simulink model "SalientPolePMSM"  (R2020b)
settings: Solver=VariableStepAuto  StartTime=0  StopTime=1  MaxStep=1e-4  RelTol=1e-4
values from neighbouring files (symbols this model uses):
  Bgain = 1    [DataSalientPolePMSM-DESKTOP-IINSHMA.m]    (also in DataSalientPolePMSM.m)
  Gcc_1ord = 1/(s/bandwidth(Gcc) + 1)    [DataSalientPolePMSM-DESKTOP-IINSHMA.m]    (also in DataSalientPolePMSM.m)
  lamdVec = mot.Ld*idVec+mot.lammg    [DataSalientPolePMSM-DESKTOP-IINSHMA.m]    (also in DataSalientPolePMSM.m)
  lamqVec = mot.Lq*iqVec    [DataSalientPolePMSM-DESKTOP-IINSHMA.m]    (also in DataSalientPolePMSM.m)
  TAB0_abc = Tabc_AB0^-1    [DataSalientPolePMSM-DESKTOP-IINSHMA.m]    (also in DataSalientPolePMSM.m)
  Tabc_AB0 = 2/3.*[     1       -1/2       -1/2 ... (first row only)    [DataSalientPolePMSM-DESKTOP-IINSHMA.m]    (also in DataSalientPolePMSM.m)
  Talphabeta_abc = Tabc_alphabeta^(-1)    [DataSalientPolePMSM-DESKTOP-IINSHMA.m]    (also in DataSalientPolePMSM.m)
undefined symbols (not defined in the file or in its folder): DiscIntNeverNeededParam, dqpll, inv, kid, kpd, magnitude, meas, mot, Obs, PI, stconv
libraries: simulink x53, pid_lib x3, powerlib x2, eeBldcCommutationLogic x1, electricdrivelib x1
(part 3 of 7)

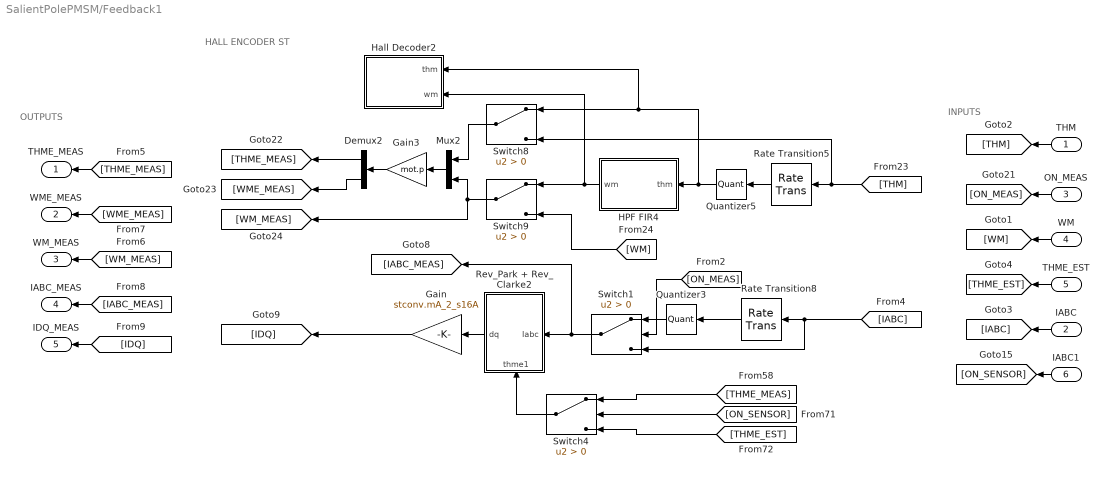
== system SalientPolePMSM/Feedback1 ==
  note: OUTPUTS
  note: INPUTS
  note: HALL ENCODER ST
  THM : Inport
  IABC : Inport  Port=2
  ON_MEAS : Inport  Port=3
  WM : Inport  Port=4
  THME_EST : Inport  Port=5
  IABC1 : Inport  Port=6
  Demux2 : Demux  Outputs=2
  Gain : Gain  Gain=stconv.mA_2_s16A
  Gain3 : Gain  Gain=mot.p
  HPF FIR4 : MATLAB Function  TreatAsAtomicUnit=on
  Hall Decoder2 : Subsystem
  Mux2 : Mux  Inputs=2
  Quantizer3 : Quantizer  QuantizationInterval=meas.cur.adc.q
  Quantizer5 : Quantizer  QuantizationInterval=meas.hall.q
  Rate Transition5 : RateTransition  OutPortSampleTime=meas.hall.Ts
  Rate Transition8 : RateTransition  OutPortSampleTime=inv.Tpwm
  Rev_Park + Rev_Clarke2 : Subsystem
      settings: PortSchema="{\"entries\":[{\"content\":{\"sides\":[{\"content\":{\"connectorIds\":[\"In1\"]},\"type\":\"ConnectorPlacement.EquallySpacedRectSide\",\"uuid\":\"2aae3f04-c402-455e-9a5d-4c573bec95dc\"},{\"content\":{\"connectorIds\":[\"Out1\"],\"side\":\"RIGHT\"},\"type\":\"ConnectorPlacement.EquallySpacedRectSide\",\"uuid\":\"f1532c60-2267-456b-9c2f-34e60e60798d\"},{\"content\":{\"connectorIds\":[],\"side\":\"TOP\"},\"type\":\"ConnectorPlacement.EquallySpacedRectSide\",\"uuid\":\"04e1a6cc-513a-47f7-a63d-759add73a2e3\"},{\"content\":{\"connectorIds\":[\"In2\"],\"side\":\"BOTTOM\"},\"type\":\"ConnectorPlacement.EquallySpacedRectSide\",\"uuid\":\"e4fadd8d-bc98-4107-9436-b30fd69f2e4f\"},{\"content\":{\"connectorIds\":[],\"side\":\"HIDDEN\"},\"type\":\"ConnectorPlacement.EquallySpacedRectSide\",\"uuid\":\"086bd472-9627-4f82-bc83-4764e9943a88\"}]},\"type\":\"ConnectorPlacement.EquallySpacedConnector\",\"uuid\":\"0de85400-6c41-4ce8-8482-fdca09eb4650\"}],\"packageUris\":[\"http://schema.mathworks.com/mf0/Connector/R2020b\"],\"version\":\"1.0\"}"
  Switch{1,4,8..9} (4 alike) : Switch  Criteria=u2 > Threshold
  THME_MEAS : Outport
  WME_MEAS : Outport  Port=2
  WM_MEAS : Outport  Port=3
  IABC_MEAS : Outport  Port=4
  IDQ_MEAS : Outport  Port=5
  wires:
  THME_EST/1 -> [THME_EST]
  WM/1 -> [WM]
  ON_MEAS/1 -> [ON_MEAS]
  Switch1/1 -> Rev_Park + Rev_Clarke2/1(Iabc), [IABC_MEAS]
  [ON_MEAS] -> Switch1/2
  Rate Transition8/1 -> Quantizer3/1
  Quantizer3/1 -> Switch1/1
  THM/1 -> [THM]
  IABC/1 -> [IABC]
  [IABC] -> Switch1/3, Rate Transition8/1
  [THME_MEAS] -> THME_MEAS/1
  [WME_MEAS] -> WME_MEAS/1
  [WM_MEAS] -> WM_MEAS/1
  [IDQ] -> IDQ_MEAS/1
  [IABC_MEAS] -> IABC_MEAS/1
  Rev_Park + Rev_Clarke2/1(dq) -> Gain/1
  IABC1/1 -> [ON_SENSOR]
  [ON_SENSOR] -> Switch4/2
  [WM] -> Switch9/3
  [THM] -> Switch8/3, Rate Transition5/1
  Demux2/2 -> [WME_MEAS]
  Mux2/1 -> Gain3/1
  Gain3/1 -> Demux2/1
  Rate Transition5/1 -> Quantizer5/1
  Switch8/1 -> Mux2/1
  HPF FIR4/1(wm) -> Switch9/1, Hall Decoder2/2(wm)
  Switch9/1 -> Mux2/2, [WM_MEAS]
  Demux2/1 -> [THME_MEAS]
  Quantizer5/1 -> HPF FIR4/1(thm), Hall Decoder2/1(thm), Switch8/1
  Gain/1 -> [IDQ]
  [THME_MEAS] -> Switch4/1
  [THME_EST] -> Switch4/3
  Switch4/1 -> Rev_Park + Rev_Clarke2/2(thme1)

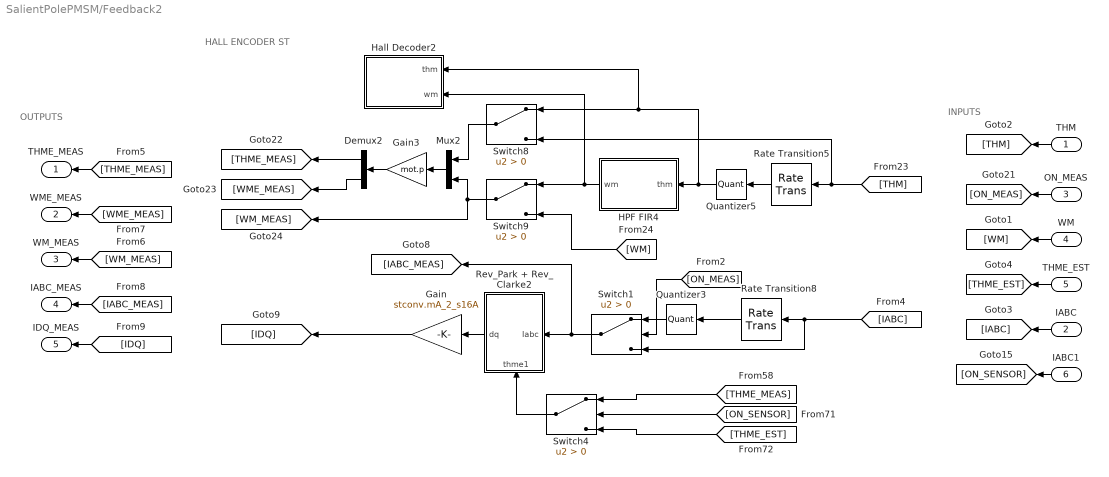
== system SalientPolePMSM/Feedback2 ==
  note: OUTPUTS
  note: INPUTS
  note: HALL ENCODER ST
  THM : Inport
  IABC : Inport  Port=2
  ON_MEAS : Inport  Port=3
  WM : Inport  Port=4
  THME_EST : Inport  Port=5
  IABC1 : Inport  Port=6
  Demux2 : Demux  Outputs=2
  Gain : Gain  Gain=stconv.mA_2_s16A
  Gain3 : Gain  Gain=mot.p
  HPF FIR4 : MATLAB Function  TreatAsAtomicUnit=on
  Hall Decoder2 : Subsystem
  Mux2 : Mux  Inputs=2
  Quantizer3 : Quantizer  QuantizationInterval=meas.cur.adc.q
  Quantizer5 : Quantizer  QuantizationInterval=meas.hall.q
  Rate Transition5 : RateTransition  OutPortSampleTime=meas.hall.Ts
  Rate Transition8 : RateTransition  OutPortSampleTime=inv.Tpwm
  Rev_Park + Rev_Clarke2 : Subsystem
      settings: PortSchema="{\"entries\":[{\"content\":{\"sides\":[{\"content\":{\"connectorIds\":[\"In1\"]},\"type\":\"ConnectorPlacement.EquallySpacedRectSide\",\"uuid\":\"2aae3f04-c402-455e-9a5d-4c573bec95dc\"},{\"content\":{\"connectorIds\":[\"Out1\"],\"side\":\"RIGHT\"},\"type\":\"ConnectorPlacement.EquallySpacedRectSide\",\"uuid\":\"f1532c60-2267-456b-9c2f-34e60e60798d\"},{\"content\":{\"connectorIds\":[],\"side\":\"TOP\"},\"type\":\"ConnectorPlacement.EquallySpacedRectSide\",\"uuid\":\"04e1a6cc-513a-47f7-a63d-759add73a2e3\"},{\"content\":{\"connectorIds\":[\"In2\"],\"side\":\"BOTTOM\"},\"type\":\"ConnectorPlacement.EquallySpacedRectSide\",\"uuid\":\"e4fadd8d-bc98-4107-9436-b30fd69f2e4f\"},{\"content\":{\"connectorIds\":[],\"side\":\"HIDDEN\"},\"type\":\"ConnectorPlacement.EquallySpacedRectSide\",\"uuid\":\"086bd472-9627-4f82-bc83-4764e9943a88\"}]},\"type\":\"ConnectorPlacement.EquallySpacedConnector\",\"uuid\":\"0de85400-6c41-4ce8-8482-fdca09eb4650\"}],\"packageUris\":[\"http://schema.mathworks.com/mf0/Connector/R2020b\"],\"version\":\"1.0\"}"
  Switch{1,4,8..9} (4 alike) : Switch  Criteria=u2 > Threshold
  THME_MEAS : Outport
  WME_MEAS : Outport  Port=2
  WM_MEAS : Outport  Port=3
  IABC_MEAS : Outport  Port=4
  IDQ_MEAS : Outport  Port=5
  wires:
  THME_EST/1 -> [THME_EST]
  WM/1 -> [WM]
  ON_MEAS/1 -> [ON_MEAS]
  Switch1/1 -> Rev_Park + Rev_Clarke2/1(Iabc), [IABC_MEAS]
  [ON_MEAS] -> Switch1/2
  Rate Transition8/1 -> Quantizer3/1
  Quantizer3/1 -> Switch1/1
  THM/1 -> [THM]
  IABC/1 -> [IABC]
  [IABC] -> Switch1/3, Rate Transition8/1
  [THME_MEAS] -> THME_MEAS/1
  [WME_MEAS] -> WME_MEAS/1
  [WM_MEAS] -> WM_MEAS/1
  [IDQ] -> IDQ_MEAS/1
  [IABC_MEAS] -> IABC_MEAS/1
  Rev_Park + Rev_Clarke2/1(dq) -> Gain/1
  IABC1/1 -> [ON_SENSOR]
  [ON_SENSOR] -> Switch4/2
  [WM] -> Switch9/3
  [THM] -> Switch8/3, Rate Transition5/1
  Demux2/2 -> [WME_MEAS]
  Mux2/1 -> Gain3/1
  Gain3/1 -> Demux2/1
  Rate Transition5/1 -> Quantizer5/1
  Switch8/1 -> Mux2/1
  HPF FIR4/1(wm) -> Switch9/1, Hall Decoder2/2(wm)
  Switch9/1 -> Mux2/2, [WM_MEAS]
  Demux2/1 -> [THME_MEAS]
  Quantizer5/1 -> HPF FIR4/1(thm), Hall Decoder2/1(thm), Switch8/1
  Gain/1 -> [IDQ]
  [THME_MEAS] -> Switch4/1
  [THME_EST] -> Switch4/3
  Switch4/1 -> Rev_Park + Rev_Clarke2/2(thme1)

== system SalientPolePMSM/Fuzzy PI ==
  note: INPUTS:
  note: OUTPUT:
  wm* : Inport
  wm : Inport  Port=2
  " " : MATLAB Function  TreatAsAtomicUnit=on
  "  " : MATLAB Function  TreatAsAtomicUnit=on
  "   " : MATLAB Function  TreatAsAtomicUnit=on
  Gain : Gain  Gain=60/(2*3.14)
  Gain1 : Gain  Gain=60/(2*3.14)
  Rule base : MATLAB Function  Commented=on  TreatAsAtomicUnit=on
  Saturation : Saturate  UpperLimit=mot.IN*mot.kTau  LowerLimit=-mot.IN*mot.kTau
  Scope : Scope  NumInputPorts=2
  Scope1 : Scope  NumInputPorts=2
  Sum : Sum  Inputs=|+-
  tau*sat : Outport
  wires:
  "  "/1(isMember) -> Scope1/1, "   "/1(isMember)
  " "/1(isMember_P) -> "  "/1(isMember_P)
  Sum/1 -> " "/1(err)
  Rule base/1(y) -> ?
  " "/4(isNotMember_I) -> "  "/4(isNotMember_I)
  "  "/2(isNotMember) -> Scope1/2, "   "/2(isNotMember)
  " "/2(isNotMember_P) -> "  "/2(isNotMember_P)
  " "/3(isMember_I) -> "  "/3(isMember_I)
  wm*/1 -> Gain/1
  wm/1 -> Gain1/1
  Gain/1 -> Sum/1
  Gain1/1 -> Sum/2
  "   "/1(tau) -> tau*sat/1

== system SalientPolePMSM/Fuzzy PI1 ==
  note: INPUTS:
  note: OUTPUT:
  wm* : Inport
  wm : Inport  Port=2
  " " : MATLAB Function  TreatAsAtomicUnit=on
  "  " : MATLAB Function  TreatAsAtomicUnit=on
  "   " : MATLAB Function  TreatAsAtomicUnit=on
  Rule base : MATLAB Function  Commented=on  TreatAsAtomicUnit=on
  Saturation : Saturate  UpperLimit=10  LowerLimit=-10
  Scope : Scope  NumInputPorts=2
  Scope1 : Scope  NumInputPorts=2
  Sum : Sum  Inputs=|+-
  tau*sat : Outport
  wires:
  "  "/1(isMember) -> Scope1/1, "   "/1(isMember)
  " "/1(isMember_P) -> "  "/1(isMember_P)
  Sum/1 -> " "/1(err)
  Rule base/1(y) -> ?
  " "/4(isNotMember_I) -> "  "/4(isNotMember_I)
  "  "/2(isNotMember) -> Scope1/2, "   "/2(isNotMember)
  " "/2(isNotMember_P) -> "  "/2(isNotMember_P)
  " "/3(isMember_I) -> "  "/3(isMember_I)
  wm*/1 -> Scope/1, Sum/1
  wm/1 -> Scope/2, Sum/2
  Saturation/1 -> tau*sat/1  "tau*sat"
  "   "/1(tau) -> Saturation/1  "tau*"

== system SalientPolePMSM/Fuzzy PI2 ==
  note: INPUTS:
  note: OUTPUT:
  wm* : Inport
  wm : Inport  Port=2
  " " : MATLAB Function  TreatAsAtomicUnit=on
  "  " : MATLAB Function  TreatAsAtomicUnit=on
  "   " : MATLAB Function  TreatAsAtomicUnit=on
  Gain : Gain  Gain=60/(2*3.14)
  Gain1 : Gain  Gain=60/(2*3.14)
  Rule base : MATLAB Function  Commented=on  TreatAsAtomicUnit=on
  Saturation : Saturate  UpperLimit=mot.IN*mot.kTau  LowerLimit=-mot.IN*mot.kTau
  Scope : Scope  NumInputPorts=2
  Scope1 : Scope  NumInputPorts=2
  Sum : Sum  Inputs=|+-
  tau*sat : Outport
  wires:
  "  "/1(isMember) -> Scope1/1, "   "/1(isMember)
  " "/1(isMember_P) -> "  "/1(isMember_P)
  Sum/1 -> " "/1(err)
  Rule base/1(y) -> ?
  " "/4(isNotMember_I) -> "  "/4(isNotMember_I)
  "  "/2(isNotMember) -> Scope1/2, "   "/2(isNotMember)
  " "/2(isNotMember_P) -> "  "/2(isNotMember_P)
  " "/3(isMember_I) -> "  "/3(isMember_I)
  wm*/1 -> Gain/1
  wm/1 -> Gain1/1
  Gain/1 -> Sum/1
  Gain1/1 -> Sum/2
  "   "/1(tau) -> tau*sat/1

== system SalientPolePMSM/INVERTER ==
  note: INPUTS:
  note: OUTPUTS:
  uAB : Inport
  uBus : Inport  Port=2
  iabc : Inport  Port=3
  INVERTER power driver : Subsystem
  SVM algorithm : Subsystem
  uabc_n* : Outport
  uabc_n*nonideal : Outport  Port=2
  satON : Outport  Port=3
  duties : Outport  Port=4
  wires:
  uBus/1 -> SVM algorithm/2(uBus), INVERTER power driver/2(uBus)
  SVM algorithm/2(satON) -> [satON]
  [satON] -> satON/1
  SVM algorithm/1(duties) -> duties/1, INVERTER power driver/1(duties)  "duties"
  iabc/1 -> INVERTER power driver/3(iabc)
  INVERTER power driver/1(uabc_n*) -> uabc_n*/1
  INVERTER power driver/2(uabc_n*nonideal) -> uabc_n*nonideal/1
  uAB/1 -> SVM algorithm/1(UABref)

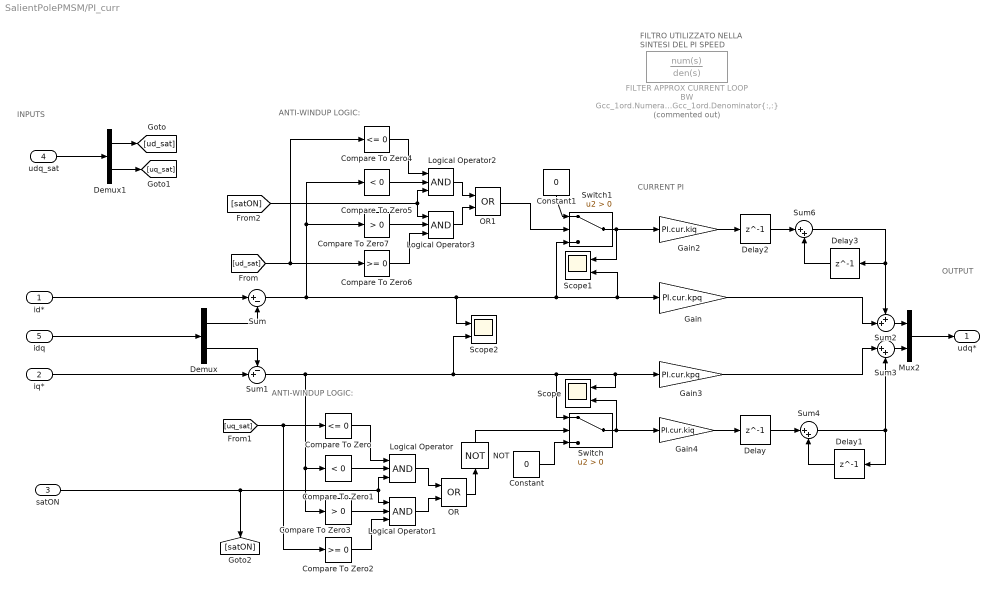
== system SalientPolePMSM/PI_curr ==
  note: FILTRO UTILIZZATO
      | NELLA SINTESI DEL
      | PI SPEED
  note: CURRENT PI
  note: ANTI-WINDUP LOGIC:
  note: ANTI-WINDUP LOGIC:
  note: OUTPUT
  note: INPUTS
  id* : Inport
  iq* : Inport  Port=2
  satON : Inport  Port=3
  udq_sat : Inport  Port=4
  idq : Inport  Port=5
  Compare To Zero : simulink/Logic and Bit Operations/Compare To Zero  relop=<=  OutDataTypeStr=boolean  ZeroCross=off
  Compare To Zero1 : simulink/Logic and Bit Operations/Compare To Zero  relop=<  OutDataTypeStr=boolean  ZeroCross=off
  Compare To Zero2 : simulink/Logic and Bit Operations/Compare To Zero  relop=>=  OutDataTypeStr=boolean  ZeroCross=off
  Compare To Zero3 : simulink/Logic and Bit Operations/Compare To Zero  relop=>  OutDataTypeStr=boolean  ZeroCross=off
  Compare To Zero4 : simulink/Logic and Bit Operations/Compare To Zero  relop=<=  OutDataTypeStr=boolean  ZeroCross=off
  Compare To Zero5 : simulink/Logic and Bit Operations/Compare To Zero  relop=<  OutDataTypeStr=boolean  ZeroCross=off
  Compare To Zero6 : simulink/Logic and Bit Operations/Compare To Zero  relop=>=  OutDataTypeStr=boolean  ZeroCross=off
  Compare To Zero7 : simulink/Logic and Bit Operations/Compare To Zero  relop=>  OutDataTypeStr=boolean  ZeroCross=off
  Constant : Constant  Value=0
  Constant1 : Constant  Value=0
  Delay{,1..3} (4 alike) : Delay  DelayLength=1  SampleTime=PI.cur.Ts
  Demux : Demux  Outputs=2
  Demux1 : Demux  Outputs=2
  FILTER APPROX CURRENT LOOP BW : TransferFcn  Commented=on  Numerator=Gcc_1ord.Numerator{:,:}  Denominator=Gcc_1ord.Denominator{:,:}
  Gain : Gain  Gain=PI.cur.kpq
  Gain2 : Gain  Gain=PI.cur.kiq
  Gain3 : Gain  Gain=PI.cur.kpq
  Gain4 : Gain  Gain=PI.cur.kiq
  Logical Operator{,1..3} (4 alike) : Logic  Inputs=3  AllPortsSameDT=off  OutDataTypeStr=boolean
  Mux2 : Mux  Inputs=2
  NOT : Logic  Operator=NOT  AllPortsSameDT=off  OutDataTypeStr=boolean
  OR : Logic  Operator=OR  AllPortsSameDT=off  OutDataTypeStr=boolean
  OR1 : Logic  Operator=OR  AllPortsSameDT=off  OutDataTypeStr=boolean
  Scope : Scope  NumInputPorts=2
  Scope1 : Scope  NumInputPorts=2
  Scope2 : Scope  NumInputPorts=2
  Sum : Sum  Inputs=|+-
  Sum1 : Sum  Inputs=-+|
  Sum2 : Sum  Inputs=++|
  Sum3 : Sum  Inputs=|++
  Sum4 : Sum  Inputs=|++
  Sum6 : Sum  Inputs=|++
  Switch : Switch  Criteria=u2 > Threshold
  Switch1 : Switch  Criteria=u2 > Threshold
  udq* : Outport
  wires:
  Demux/2 -> Sum1/1
  Mux2/1 -> udq*/1
  Sum3/1 -> Mux2/2
  Demux/1 -> Sum/2
  Sum2/1 -> Mux2/1
  Sum4/1 -> Delay1/1, Sum3/2
  Sum1/1 -> Scope2/2, Switch/1, Scope/1, Gain3/1, Compare To Zero3/1, Compare To Zero1/1
  Gain/1 -> Sum2/2
  Gain4/1 -> Delay/1
  Gain3/1 -> Sum3/1
  idq/1 -> Demux/1
  id*/1 -> Sum/1
  Switch/1 -> Scope/2, Gain4/1
  Constant/1 -> Switch/3
  OR/1 -> NOT/1
  NOT/1 -> Switch/2
  satON/1 -> [satON], Logical Operator/3, Logical Operator1/1
  Logical Operator/1 -> OR/1
  Logical Operator1/1 -> OR/2
  Compare To Zero1/1 -> Logical Operator/2
  Compare To Zero/1 -> Logical Operator/1
  Compare To Zero2/1 -> Logical Operator1/3
  [uq_sat] -> Compare To Zero2/1, Compare To Zero/1
  Compare To Zero3/1 -> Logical Operator1/2
  Compare To Zero7/1 -> Logical Operator3/2
  [ud_sat] -> Compare To Zero4/1, Compare To Zero6/1
  Compare To Zero6/1 -> Logical Operator3/3
  Compare To Zero4/1 -> Logical Operator2/1
  Compare To Zero5/1 -> Logical Operator2/2
  Logical Operator3/1 -> OR1/2
  Logical Operator2/1 -> OR1/1
  [satON] -> Logical Operator2/3, Logical Operator3/1
  OR1/1 -> Switch1/2
  Constant1/1 -> Switch1/1
  Sum/1 -> Scope2/1, Scope1/2, Gain/1, Switch1/3, Compare To Zero7/1, Compare To Zero5/1
  Switch1/1 -> Scope1/1, Gain2/1
  udq_sat/1 -> Demux1/1
  Demux1/1 -> [ud_sat]
  Demux1/2 -> [uq_sat]
  iq*/1 -> Sum1/2
  Delay/1 -> Sum4/1
  Delay1/1 -> Sum4/2
  Delay3/1 -> Sum6/2
  Delay2/1 -> Sum6/1
  Sum6/1 -> Delay3/1, Sum2/1
  Gain2/1 -> Delay2/1

== system SalientPolePMSM/PI_speed ==
  note: OUTPUT:
  note: INPUTS:
  wm* : Inport
  wm : Inport  Port=2
  Delay : Delay  DelayLength=1  SampleTime=PI.vel.Ts
  Delay1 : Delay  DelayLength=1  SampleTime=PI.vel.Ts
  Delay2 : Delay  DelayLength=1  SampleTime=PI.vel.Ts
  Gain2 : Gain  Gain=PI.vel.kt
  Gain3 : Gain  Gain=PI.vel.kp
  Gain4 : Gain  Gain=PI.vel.ki
  Saturation : Saturate  UpperLimit=mot.IN*mot.kTau  LowerLimit=-mot.IN*mot.kTau
  Scope : Scope  NumInputPorts=2
  Sum : Sum  Inputs=|+-
  Sum1 : Sum  Inputs=|+-
  Sum2 : Sum  Inputs=+|-
  Sum3 : Sum  Inputs=|++
  Sum4 : Sum  Inputs=|++
  tau*sat : Outport
  wires:
  Saturation/1 -> tau*sat/1, Sum2/2  "tau*sat"
  Gain2/1 -> Sum1/2
  Gain3/1 -> Sum3/1
  Sum3/1 -> Sum2/1, Saturation/1  "tau*"
  Sum/1 -> Gain4/1, Gain3/1
  Sum2/1 -> Delay2/1
  Gain4/1 -> Sum1/1
  wm*/1 -> Scope/1, Sum/1
  wm/1 -> Scope/2, Sum/2
  Delay/1 -> Sum4/1
  Sum4/1 -> Sum3/2, Delay1/1
  Delay1/1 -> Sum4/2
  Sum1/1 -> Delay/1
  Delay2/1 -> Gain2/1

== system SalientPolePMSM/PI_speed1 ==
  note: OUTPUT:
  note: INPUTS:
  wm* : Inport
  wm : Inport  Port=2
  Delay : Delay  DelayLength=1  SampleTime=PI.vel.Ts
  Delay1 : Delay  DelayLength=1  SampleTime=PI.vel.Ts
  Delay2 : Delay  DelayLength=1  SampleTime=PI.vel.Ts
  Gain : Gain  Gain=60/(2*3.14)
  Gain1 : Gain  Gain=60/(2*3.14)
  Gain2 : Gain  Gain=PI.vel.kt
  Gain3 : Gain  Gain=PI.vel.kp
  Gain4 : Gain  Gain=PI.vel.ki
  Saturation : Saturate  UpperLimit=mot.IN*1000  LowerLimit=-mot.IN*1000
  Scope : Scope  NumInputPorts=2
  Sum : Sum  Inputs=|+-
  Sum1 : Sum  Inputs=|+-
  Sum2 : Sum  Inputs=+|-
  Sum3 : Sum  Inputs=|++
  Sum4 : Sum  Inputs=|++
  tau*sat : Outport
  wires:
  Gain3/1 -> Sum3/1
  Sum/1 -> Gain4/1, Gain3/1
  Gain4/1 -> Sum1/1
  Delay/1 -> Sum4/1
  Sum4/1 -> Sum3/2, Delay1/1
  Delay1/1 -> Sum4/2
  Sum1/1 -> Delay/1
  Delay2/1 -> Gain2/1
  Sum2/1 -> Delay2/1
  Gain2/1 -> Sum1/2
  wm/1 -> Gain1/1
  wm*/1 -> Gain/1
  Gain/1 -> Sum/1
  Gain1/1 -> Sum/2
  Sum3/1 -> tau*sat/1  "tau*"

== system SalientPolePMSM/PI_speed2 ==
  note: OUTPUT:
  note: INPUTS:
  wm* : Inport
  wm : Inport  Port=2
  Delay : Delay  DelayLength=1  SampleTime=PI.vel.Ts
  Delay1 : Delay  DelayLength=1  SampleTime=PI.vel.Ts
  Delay2 : Delay  DelayLength=1  SampleTime=PI.vel.Ts
  Gain2 : Gain  Gain=0.040/10
  Gain3 : Gain  Gain=10
  Gain4 : Gain  Gain=0.040
  Saturation : Saturate  UpperLimit=10  LowerLimit=-10
  Scope : Scope  NumInputPorts=2
  Sum : Sum  Inputs=|+-
  Sum1 : Sum  Inputs=|+-
  Sum2 : Sum  Inputs=+|-
  Sum3 : Sum  Inputs=|++
  Sum4 : Sum  Inputs=|++
  tau*sat : Outport
  wires:
  Saturation/1 -> Sum2/2, tau*sat/1  "tau*sat"
  Gain3/1 -> Sum3/1
  Sum3/1 -> Sum2/1, Saturation/1  "tau*"
  Sum/1 -> Gain4/1, Gain3/1
  Sum2/1 -> Delay2/1
  Gain4/1 -> Sum1/1
  wm*/1 -> Scope/1, Sum/1
  wm/1 -> Scope/2, Sum/2
  Delay/1 -> Sum4/1
  Sum4/1 -> Sum3/2, Delay1/1
  Delay1/1 -> Sum4/2
  Sum1/1 -> Delay/1
  Delay2/1 -> Gain2/1
  Gain2/1 -> Sum1/2

== system SalientPolePMSM/PI_speed3 ==
  note: OUTPUT:
  note: INPUTS:
  wm* : Inport
  wm : Inport  Port=2
  Delay : Delay  DelayLength=1  SampleTime=PI.vel.Ts
  Delay1 : Delay  DelayLength=1  SampleTime=PI.vel.Ts
  Delay2 : Delay  DelayLength=1  SampleTime=PI.vel.Ts
  Gain : Gain  Gain=60/(2*3.14)
  Gain1 : Gain  Gain=60/(2*3.14)
  Gain2 : Gain  Gain=PI.vel.kt
  Gain3 : Gain  Gain=PI.vel.kp
  Gain4 : Gain  Gain=PI.vel.ki
  Saturation : Saturate  UpperLimit=mot.IN*1000  LowerLimit=-mot.IN*1000
  Scope : Scope  NumInputPorts=2
  Sum : Sum  Inputs=|+-
  Sum1 : Sum  Inputs=|+-
  Sum2 : Sum  Inputs=+|-
  Sum3 : Sum  Inputs=|++
  Sum4 : Sum  Inputs=|++
  tau*sat : Outport
  wires:
  Gain3/1 -> Sum3/1
  Sum/1 -> Gain4/1, Gain3/1
  Gain4/1 -> Sum1/1
  Delay/1 -> Sum4/1
  Sum4/1 -> Sum3/2, Delay1/1
  Delay1/1 -> Sum4/2
  Sum1/1 -> Delay/1
  Delay2/1 -> Gain2/1
  Sum2/1 -> Delay2/1
  Gain2/1 -> Sum1/2
  wm/1 -> Gain1/1
  wm*/1 -> Gain/1
  Gain/1 -> Sum/1
  Gain1/1 -> Sum/2
  Sum3/1 -> tau*sat/1  "tau*"

== system SalientPolePMSM/SENSORLESS ALGORITHM ==
  iabc : Inport
  uabc : Inport  Port=2
  ON_approx : Inport  Port=3
  ADD_integrator : Inport  Port=4
  DECOUPLING : Subsystem
      settings: PortSchema="{\"entries\":[{\"content\":{\"sides\":[{\"content\":{\"connectorIds\":[\"In1\",\"In2\"]},\"type\":\"ConnectorPlacement.EquallySpacedRectSide\",\"uuid\":\"11caacf5-0bb5-4a8d-b3e9-7b1e88488e40\"},{\"content\":{\"connectorIds\":[\"Out1\",\"Out2\"],\"side\":\"RIGHT\"},\"type\":\"ConnectorPlacement.EquallySpacedRectSide\",\"uuid\":\"6263df69-80cd-4b04-a89b-dfca9161a93e\"},{\"content\":{\"connectorIds\":[],\"side\":\"TOP\"},\"type\":\"ConnectorPlacement.EquallySpacedRectSide\",\"uuid\":\"898c91db-8461-4171-8db9-87a99b66ce40\"},{\"content\":{\"connectorIds\":[\"In3\"],\"side\":\"BOTTOM\"},\"type\":\"ConnectorPlacement.EquallySpacedRectSide\",\"uuid\":\"185c1e28-6dbc-44e9-9bab-ce833de258e7\"},{\"content\":{\"connectorIds\":[],\"side\":\"HIDDEN\"},\"type\":\"ConnectorPlacement.EquallySpacedRectSide\",\"uuid\":\"0f2378b2-18e5-4bfa-bdaa-e448fe90a90d\"}]},\"type\":\"ConnectorPlacement.EquallySpacedConnector\",\"uuid\":\"5ac053f8-067e-460f-b603-fa451a6d3395\"}],\"packageUris\":[\"http://schema.mathworks.com/mf0/Connector/R2020b\"],\"version\":\"1.0\"}"
  Demux : Demux  Outputs=2
  Demux1 : Demux  Outputs=2
  Demux2 : Demux  Outputs=2
  ESTIMETOR ed : Subsystem
  ESTIMETOR eq : Subsystem
  Integrator1 : Integrator
  PI : Subsystem
  PII : Subsystem
  Rate Transition{1,4..7} (5 alike) : RateTransition
  Subsystem1 : Subsystem
      settings: PortSchema="{\"entries\":[{\"content\":{\"sides\":[{\"content\":{\"connectorIds\":[\"In1\"]},\"type\":\"ConnectorPlacement.EquallySpacedRectSide\",\"uuid\":\"4ed90ab9-1fa1-426e-9a51-633f86eaed93\"},{\"content\":{\"connectorIds\":[\"Out1\"],\"side\":\"RIGHT\"},\"type\":\"ConnectorPlacement.EquallySpacedRectSide\",\"uuid\":\"a783641a-eefd-4804-96bc-e093b09f1b23\"},{\"content\":{\"connectorIds\":[\"In2\"],\"side\":\"TOP\"},\"type\":\"ConnectorPlacement.EquallySpacedRectSide\",\"uuid\":\"b71fad55-6d7c-4fa9-b8c9-7c2d781b5980\"},{\"content\":{\"connectorIds\":[],\"side\":\"BOTTOM\"},\"type\":\"ConnectorPlacement.EquallySpacedRectSide\",\"uuid\":\"0ef0ee48-37c5-4f1f-a4a0-75388778f62a\"},{\"content\":{\"connectorIds\":[],\"side\":\"HIDDEN\"},\"type\":\"ConnectorPlacement.EquallySpacedRectSide\",\"uuid\":\"d9128c0c-5cc0-40ee-9c52-e819b4b0207f\"}]},\"type\":\"ConnectorPlacement.EquallySpacedConnector\",\"uuid\":\"84170b20-7cd7-4bfe-ad20-891cbad09232\"}],\"packageUris\":[\"http://schema.mathworks.com/mf0/Connector/R2020b\"],\"version\":\"1.0\"}"
  Subsystem2 : Subsystem
      settings: PortSchema="{\"entries\":[{\"content\":{\"sides\":[{\"content\":{\"connectorIds\":[\"In1\"]},\"type\":\"ConnectorPlacement.EquallySpacedRectSide\",\"uuid\":\"4ed90ab9-1fa1-426e-9a51-633f86eaed93\"},{\"content\":{\"connectorIds\":[\"Out1\"],\"side\":\"RIGHT\"},\"type\":\"ConnectorPlacement.EquallySpacedRectSide\",\"uuid\":\"a783641a-eefd-4804-96bc-e093b09f1b23\"},{\"content\":{\"connectorIds\":[],\"side\":\"TOP\"},\"type\":\"ConnectorPlacement.EquallySpacedRectSide\",\"uuid\":\"b71fad55-6d7c-4fa9-b8c9-7c2d781b5980\"},{\"content\":{\"connectorIds\":[\"In2\"],\"side\":\"BOTTOM\"},\"type\":\"ConnectorPlacement.EquallySpacedRectSide\",\"uuid\":\"0ef0ee48-37c5-4f1f-a4a0-75388778f62a\"},{\"content\":{\"connectorIds\":[],\"side\":\"HIDDEN\"},\"type\":\"ConnectorPlacement.EquallySpacedRectSide\",\"uuid\":\"d9128c0c-5cc0-40ee-9c52-e819b4b0207f\"}]},\"type\":\"ConnectorPlacement.EquallySpacedConnector\",\"uuid\":\"84170b20-7cd7-4bfe-ad20-891cbad09232\"}],\"packageUris\":[\"http://schema.mathworks.com/mf0/Connector/R2020b\"],\"version\":\"1.0\"}"
  Switch : Switch  Criteria=u2 > Threshold
  Switch1 : Switch  Criteria=u2 > Threshold
  Terminator : Terminator
  Transfer Fcn : TransferFcn  Numerator=[dqpll.lpf.Bc]  Denominator=[1 dqpll.lpf.Bc]
  atan : MATLAB Function  TreatAsAtomicUnit=on
  atanApprox : MATLAB Function  TreatAsAtomicUnit=on
  thme_est : Outport
  wme_est : Outport  Port=2
  wires:
  Switch1/1 -> Integrator1/1, Transfer Fcn/1
  Demux1/1 -> ESTIMETOR eq/1(uq)
  Demux1/2 -> ESTIMETOR eq/2(iq)
  Demux2/1 -> ESTIMETOR ed/1(ud)
  Demux2/2 -> ESTIMETOR ed/2(id)
  atanApprox/1(thme) -> Switch/1
  Subsystem2/1(dq) -> DECOUPLING/2(udq_est)
  Subsystem1/1(dq) -> Demux/1, DECOUPLING/1(idq_est)
  DECOUPLING/1(ud' id) -> Demux2/1
  Transfer Fcn/1 -> Rate Transition1/1, DECOUPLING/3(wme_est), Rate Transition5/1
  Integrator1/1 -> [THME_EST], Rate Transition4/1
  DECOUPLING/2(uq' iq) -> Demux1/1
  ESTIMETOR eq/1(eq) -> atan/2(eq)
  ON_approx/1 -> Switch/2
  Demux/2 -> Terminator/1
  [THME_EST] -> Subsystem1/2(thme), Subsystem2/2(thme)
  Switch/1 -> PII/1(e), PI/1(e)
  Demux/1 -> atanApprox/1(id)
  ESTIMETOR ed/1(ed) -> atanApprox/2(ed), atan/1(ed)
  iabc/1 -> Rate Transition6/1
  Rate Transition4/1 -> thme_est/1
  Rate Transition7/1 -> Subsystem2/1(abc)
  Rate Transition5/1 -> wme_est/1
  Rate Transition6/1 -> Subsystem1/1(abc)
  uabc/1 -> Rate Transition7/1
  atan/1(thme) -> Switch/3
  Rate Transition1/1 -> atanApprox/3(wme_est)
  ADD_integrator/1 -> Switch1/2
  PII/1(w_est) -> Switch1/1
  PI/1(w_est) -> Switch1/3

== system SalientPolePMSM/SENSORLESS ALGORITHM1 ==
  iabc : Inport
  uabc : Inport  Port=2
  ON_approx : Inport  Port=3
  ADD_integrator : Inport  Port=4
  DECOUPLING : Subsystem
      settings: PortSchema="{\"entries\":[{\"content\":{\"sides\":[{\"content\":{\"connectorIds\":[\"In1\",\"In2\"]},\"type\":\"ConnectorPlacement.EquallySpacedRectSide\",\"uuid\":\"11caacf5-0bb5-4a8d-b3e9-7b1e88488e40\"},{\"content\":{\"connectorIds\":[\"Out1\",\"Out2\"],\"side\":\"RIGHT\"},\"type\":\"ConnectorPlacement.EquallySpacedRectSide\",\"uuid\":\"6263df69-80cd-4b04-a89b-dfca9161a93e\"},{\"content\":{\"connectorIds\":[],\"side\":\"TOP\"},\"type\":\"ConnectorPlacement.EquallySpacedRectSide\",\"uuid\":\"898c91db-8461-4171-8db9-87a99b66ce40\"},{\"content\":{\"connectorIds\":[\"In3\"],\"side\":\"BOTTOM\"},\"type\":\"ConnectorPlacement.EquallySpacedRectSide\",\"uuid\":\"185c1e28-6dbc-44e9-9bab-ce833de258e7\"},{\"content\":{\"connectorIds\":[],\"side\":\"HIDDEN\"},\"type\":\"ConnectorPlacement.EquallySpacedRectSide\",\"uuid\":\"0f2378b2-18e5-4bfa-bdaa-e448fe90a90d\"}]},\"type\":\"ConnectorPlacement.EquallySpacedConnector\",\"uuid\":\"5ac053f8-067e-460f-b603-fa451a6d3395\"}],\"packageUris\":[\"http://schema.mathworks.com/mf0/Connector/R2020b\"],\"version\":\"1.0\"}"
  Demux : Demux  Outputs=2
  Demux1 : Demux  Outputs=2
  Demux2 : Demux  Outputs=2
  ESTIMETOR ed : Subsystem
  ESTIMETOR eq : Subsystem
  Integrator1 : Integrator
  PI : Subsystem
  PII : Subsystem
  Rate Transition{1,4..7} (5 alike) : RateTransition
  Subsystem1 : Subsystem
      settings: PortSchema="{\"entries\":[{\"content\":{\"sides\":[{\"content\":{\"connectorIds\":[\"In1\"]},\"type\":\"ConnectorPlacement.EquallySpacedRectSide\",\"uuid\":\"4ed90ab9-1fa1-426e-9a51-633f86eaed93\"},{\"content\":{\"connectorIds\":[\"Out1\"],\"side\":\"RIGHT\"},\"type\":\"ConnectorPlacement.EquallySpacedRectSide\",\"uuid\":\"a783641a-eefd-4804-96bc-e093b09f1b23\"},{\"content\":{\"connectorIds\":[\"In2\"],\"side\":\"TOP\"},\"type\":\"ConnectorPlacement.EquallySpacedRectSide\",\"uuid\":\"b71fad55-6d7c-4fa9-b8c9-7c2d781b5980\"},{\"content\":{\"connectorIds\":[],\"side\":\"BOTTOM\"},\"type\":\"ConnectorPlacement.EquallySpacedRectSide\",\"uuid\":\"0ef0ee48-37c5-4f1f-a4a0-75388778f62a\"},{\"content\":{\"connectorIds\":[],\"side\":\"HIDDEN\"},\"type\":\"ConnectorPlacement.EquallySpacedRectSide\",\"uuid\":\"d9128c0c-5cc0-40ee-9c52-e819b4b0207f\"}]},\"type\":\"ConnectorPlacement.EquallySpacedConnector\",\"uuid\":\"84170b20-7cd7-4bfe-ad20-891cbad09232\"}],\"packageUris\":[\"http://schema.mathworks.com/mf0/Connector/R2020b\"],\"version\":\"1.0\"}"
  Subsystem2 : Subsystem
      settings: PortSchema="{\"entries\":[{\"content\":{\"sides\":[{\"content\":{\"connectorIds\":[\"In1\"]},\"type\":\"ConnectorPlacement.EquallySpacedRectSide\",\"uuid\":\"4ed90ab9-1fa1-426e-9a51-633f86eaed93\"},{\"content\":{\"connectorIds\":[\"Out1\"],\"side\":\"RIGHT\"},\"type\":\"ConnectorPlacement.EquallySpacedRectSide\",\"uuid\":\"a783641a-eefd-4804-96bc-e093b09f1b23\"},{\"content\":{\"connectorIds\":[],\"side\":\"TOP\"},\"type\":\"ConnectorPlacement.EquallySpacedRectSide\",\"uuid\":\"b71fad55-6d7c-4fa9-b8c9-7c2d781b5980\"},{\"content\":{\"connectorIds\":[\"In2\"],\"side\":\"BOTTOM\"},\"type\":\"ConnectorPlacement.EquallySpacedRectSide\",\"uuid\":\"0ef0ee48-37c5-4f1f-a4a0-75388778f62a\"},{\"content\":{\"connectorIds\":[],\"side\":\"HIDDEN\"},\"type\":\"ConnectorPlacement.EquallySpacedRectSide\",\"uuid\":\"d9128c0c-5cc0-40ee-9c52-e819b4b0207f\"}]},\"type\":\"ConnectorPlacement.EquallySpacedConnector\",\"uuid\":\"84170b20-7cd7-4bfe-ad20-891cbad09232\"}],\"packageUris\":[\"http://schema.mathworks.com/mf0/Connector/R2020b\"],\"version\":\"1.0\"}"
  Switch : Switch  Criteria=u2 > Threshold
  Switch1 : Switch  Criteria=u2 > Threshold
  Terminator : Terminator
  Transfer Fcn : TransferFcn  Numerator=[dqpll.lpf.Bc]  Denominator=[1 dqpll.lpf.Bc]
  atan : MATLAB Function  TreatAsAtomicUnit=on
  atanApprox : MATLAB Function  TreatAsAtomicUnit=on
  thme_est : Outport
  wme_est : Outport  Port=2
  wires:
  Switch1/1 -> Integrator1/1, Transfer Fcn/1
  Demux1/1 -> ESTIMETOR eq/1(uq)
  Demux1/2 -> ESTIMETOR eq/2(iq)
  Demux2/1 -> ESTIMETOR ed/1(ud)
  Demux2/2 -> ESTIMETOR ed/2(id)
  atanApprox/1(thme) -> Switch/1
  Subsystem2/1(dq) -> DECOUPLING/2(udq_est)
  Subsystem1/1(dq) -> Demux/1, DECOUPLING/1(idq_est)
  DECOUPLING/1(ud' id) -> Demux2/1
  Transfer Fcn/1 -> Rate Transition1/1, DECOUPLING/3(wme_est), Rate Transition5/1
  Integrator1/1 -> [THME_EST], Rate Transition4/1
  DECOUPLING/2(uq' iq) -> Demux1/1
  ESTIMETOR eq/1(eq) -> atan/2(eq)
  ON_approx/1 -> Switch/2
  Demux/2 -> Terminator/1
  [THME_EST] -> Subsystem1/2(thme), Subsystem2/2(thme)
  Switch/1 -> PII/1(e), PI/1(e)
  Demux/1 -> atanApprox/1(id)
  ESTIMETOR ed/1(ed) -> atanApprox/2(ed), atan/1(ed)
  iabc/1 -> Rate Transition6/1
  Rate Transition4/1 -> thme_est/1
  Rate Transition7/1 -> Subsystem2/1(abc)
  Rate Transition5/1 -> wme_est/1
  Rate Transition6/1 -> Subsystem1/1(abc)
  uabc/1 -> Rate Transition7/1
  atan/1(thme) -> Switch/3
  Rate Transition1/1 -> atanApprox/3(wme_est)
  ADD_integrator/1 -> Switch1/2
  PII/1(w_est) -> Switch1/1
  PI/1(w_est) -> Switch1/3

== system SalientPolePMSM/Subsystem ==
  In1 : Inport
  Add3 : Sum  Commented=on  Inputs=--
  Demux : Demux  Commented=on  Outputs=2
  Gain1 : Gain  Gain=TAB0_abc  Multiplication=Matrix(K*u) (u vector)
  Gain2 : Gain  Commented=on  Gain=2
  Gain3 : Gain  Commented=on  Gain=-1/sqrt(3)
  Mux2 : Mux  Commented=on  Inputs=3
  Sum1 : Sum  Commented=on  Inputs=++|
  abc : Outport
  wires:
  Add3/1 -> Mux2/3
  Demux/2 -> Gain2/1
  Gain2/1 -> Sum1/2
  Demux/1 -> Mux2/1, Add3/1, Sum1/1
  Sum1/1 -> Gain3/1
  Gain3/1 -> Mux2/2, Add3/2
  In1/1 -> Gain1/1, Demux/1
  Gain1/1 -> abc/1

== system SalientPolePMSM/Subsystem2 ==
  note: OUTPUT
  note: INPUTS
  abc : Inport
  thme : Inport  Port=2
  Add2 : Sum
  Add3 : Sum  Inputs=-+
  Cos2 : Trigonometry  Operator=cos
  Demux2 : Demux  Outputs=3
  Gain : Gain  Gain=Tabc_AB0  Multiplication=Matrix(K*u) (u vector)
  Mux1 : Mux  Inputs=2
  Product{,1..3} (4 alike) : Product
  Sin2 : Trigonometry
  Terminator : Terminator
  dq : Outport
  wires:
  Mux1/1 -> dq/1
  Sin2/1 -> Product1/2, Product2/2
  Demux2/2 -> Product3/2, Product1/1
  Product2/1 -> Add3/1
  Product3/1 -> Add3/2
  thme/1 -> Sin2/1, Cos2/1
  Demux2/1 -> Product2/1, Product/1
  Cos2/1 -> Product3/1, Product/2
  Product1/1 -> Add2/2
  Add3/1 -> Mux1/2
  Add2/1 -> Mux1/1
  Product/1 -> Add2/1
  Gain/1 -> Demux2/1  "AB0"
  Demux2/3 -> Terminator/1
  abc/1 -> Gain/1

== system SalientPolePMSM/Subsystem3 ==
  note: INPUTS
  note: OUTPUT
  dq : Inport
  thme : Inport  Port=2
  Add2 : Sum  Inputs=+-
  Add3 : Sum
  Cos2 : Trigonometry  Operator=cos
  Demux2 : Demux  Outputs=2
  Mux1 : Mux  Inputs=2
  Product{,1..3} (4 alike) : Product
  Sin2 : Trigonometry
  AB : Outport
  wires:
  dq/1 -> Demux2/1
  Product/1 -> Add2/1
  Add2/1 -> Mux1/1
  Add3/1 -> Mux1/2
  Product1/1 -> Add2/2
  Cos2/1 -> Product/2, Product3/1
  Demux2/1 -> Product/1, Product2/1
  thme/1 -> Cos2/1, Sin2/1
  Product3/1 -> Add3/2
  Product2/1 -> Add3/1
  Demux2/2 -> Product3/2, Product1/1
  Sin2/1 -> Product2/2, Product1/2
  Mux1/1 -> AB/1

== system SalientPolePMSM/Synchronous motor1 ==
  note: SPM MODEL with maps
  note: SPM MOTOR MODEL
  note: INPUTS
  note: OUTPUTS
  uabc : Inport
  tauL : Inport  Port=2
  Clarke + Park 1 : Subsystem
      settings: PortSchema="{\"entries\":[{\"content\":{\"sides\":[{\"content\":{\"connectorIds\":[\"In1\"]},\"type\":\"ConnectorPlacement.EquallySpacedRectSide\",\"uuid\":\"dfbca390-01d3-4350-a1f7-5814b855842b\"},{\"content\":{\"connectorIds\":[\"Out1\"],\"side\":\"RIGHT\"},\"type\":\"ConnectorPlacement.EquallySpacedRectSide\",\"uuid\":\"31b508dd-6a0c-4770-a977-34ff5a62a059\"},{\"content\":{\"connectorIds\":[\"In2\"],\"side\":\"TOP\"},\"type\":\"ConnectorPlacement.EquallySpacedRectSide\",\"uuid\":\"bd902134-125b-49c1-af87-7c7bfb23097c\"},{\"content\":{\"connectorIds\":[],\"side\":\"HIDDEN\"},\"type\":\"ConnectorPlacement.EquallySpacedRectSide\",\"uuid\":\"5c93052a-f73b-4726-be02-ec4253e9ca63\"}]},\"type\":\"ConnectorPlacement.EquallySpacedConnector\",\"uuid\":\"90558e66-2977-4bab-ac0f-d07dc1d3bf9d\"}],\"packageUris\":[\"http://schema.mathworks.com/mf0/Connector/R2020b\"],\"version\":\"1.0\"}"
  Constant : Constant  Value=0
  Gain1 : Gain  Gain=mot.p
  Gain2 : Gain  Gain=mot.p
  Mux : Mux  Inputs=3
  Rev_Park + Rev_Clarke : Subsystem
  SPM Motor : Subsystem
  electrical equations : Subsystem
  mechanical system : Subsystem
      settings: PortSchema="{\"entries\":[{\"content\":{\"sides\":[{\"content\":{\"connectorIds\":[\"In1\",\"In2\",\"In3\",\"In4\"]},\"type\":\"ConnectorPlacement.EquallySpacedRectSide\",\"uuid\":\"ba3eadf5-5339-4096-82c0-65ae6f7654f8\"},{\"content\":{\"connectorIds\":[\"Out1\",\"Out2\",\"Out3\"],\"side\":\"RIGHT\"},\"type\":\"ConnectorPlacement.EquallySpacedRectSide\",\"uuid\":\"5d9f567b-aeb8-4ece-a206-38434530d515\"},{\"content\":{\"connectorIds\":[\"In5\"],\"side\":\"TOP\"},\"type\":\"ConnectorPlacement.EquallySpacedRectSide\",\"uuid\":\"4d5c6e7c-fa05-44b7-bedf-9f7fec742b34\"}]},\"type\":\"ConnectorPlacement.EquallySpacedConnector\",\"uuid\":\"f68f900c-fb94-45c0-a867-bf7e311f1b8e\"}],\"packageUris\":[\"http://schema.mathworks.com/mf0/Connector/19700101\"],\"version\":\"1.0\"}"
  thm : Outport
  wm : Outport  Port=2
  taum : Outport  Port=3
  iabc : Outport  Port=4
  idq : Outport  Port=5
  theta_me : Outport  Port=6
  w_me : Outport  Port=7
  U_A : Outport  Port=8
  U_B : Outport  Port=9
  U_DQ : Outport  Port=10
  wires:
  Rev_Park + Rev_Clarke/1(abc) -> iabc/1
  Clarke + Park 1/1(dq) -> SPM Motor/1(dq)
  SPM Motor/1(theta_me) -> Clarke + Park 1/2(thme)
  Gain1/1 -> w_me/1, [WME]
  Constant/1 -> Mux/3
  [WME] -> electrical equations/3(w_me)
  [THME] -> electrical equations/2(thme)
  [THME] -> Rev_Park + Rev_Clarke/2(thme1)
  Mux/1 -> Rev_Park + Rev_Clarke/1(dq), idq/1
  electrical equations/1(lam_d) -> mechanical system/1(lam_d)
  tauL/1 -> [TAUL], mechanical system/5(tauL)
  uabc/1 -> Clarke + Park 1/1(abc), electrical equations/1(uabc)
  electrical equations/4(id) -> Mux/1, mechanical system/4(id)
  electrical equations/3(iq) -> mechanical system/3(iq), Mux/2
  electrical equations/2(lam_q) -> mechanical system/2(lam_q)
  Gain2/1 -> theta_me/1, [THME]
  SPM Motor/2(w_me) -> ?
  mechanical system/3(wm) -> wm/1, Gain1/1
  mechanical system/1(thm) -> thm/1, Gain2/1
  mechanical system/2(taum) -> taum/1
  electrical equations/5(UA) -> U_A/1
  electrical equations/6(UB) -> U_B/1
  electrical equations/7(UDQ) -> U_DQ/1

== system SalientPolePMSM/Synchronous motor2 ==
  note: OUTPUTS
  note: INPUTS
  uabc : Inport
  tauL : Inport  Port=2
  Constant : Constant  Value=0
  Gain1 : Gain  Gain=mot.p
  Gain2 : Gain  Gain=mot.p
  Mux : Mux  Inputs=3
  Scope : Scope
  Subsystem2 : Subsystem
  electrical equations : Subsystem
  mechanical system : Subsystem
      settings: PortSchema="{\"entries\":[{\"content\":{\"sides\":[{\"content\":{\"connectorIds\":[\"In1\",\"In2\",\"In3\",\"In4\"]},\"type\":\"ConnectorPlacement.EquallySpacedRectSide\",\"uuid\":\"ba3eadf5-5339-4096-82c0-65ae6f7654f8\"},{\"content\":{\"connectorIds\":[\"Out1\",\"Out2\",\"Out3\"],\"side\":\"RIGHT\"},\"type\":\"ConnectorPlacement.EquallySpacedRectSide\",\"uuid\":\"5d9f567b-aeb8-4ece-a206-38434530d515\"},{\"content\":{\"connectorIds\":[\"In5\"],\"side\":\"TOP\"},\"type\":\"ConnectorPlacement.EquallySpacedRectSide\",\"uuid\":\"4d5c6e7c-fa05-44b7-bedf-9f7fec742b34\"}]},\"type\":\"ConnectorPlacement.EquallySpacedConnector\",\"uuid\":\"f68f900c-fb94-45c0-a867-bf7e311f1b8e\"}],\"packageUris\":[\"http://schema.mathworks.com/mf0/Connector/19700101\"],\"version\":\"1.0\"}"
  thm : Outport
  wm : Outport  Port=2
  taum : Outport  Port=3
  iabc : Outport  Port=4
  wires:
  electrical equations/2(lam_q) -> mechanical system/2(lam_q)
  electrical equations/3(iq) -> Mux/2, mechanical system/3(iq)
  electrical equations/4(id) -> mechanical system/4(id), Mux/1
  uabc/1 -> Scope/1, electrical equations/1(uabc)
  mechanical system/1(thm) -> thm/1, Gain2/1
  tauL/1 -> mechanical system/5(tauL)
  mechanical system/3(wm) -> wm/1, Gain1/1
  electrical equations/1(lam_d) -> mechanical system/1(lam_d)
  Mux/1 -> Subsystem2/1(dq0)
  mechanical system/2(taum) -> taum/1
  Subsystem2/1(abc) -> iabc/1
  [THME] -> Subsystem2/2(thme)
  [THME] -> electrical equations/2(thme)
  [WME] -> electrical equations/3(w_me)
  Constant/1 -> Mux/3
  Gain1/1 -> [WME]
  Gain2/1 -> [THME]

== system SalientPolePMSM/Synchronous motor3 ==
  note: SPM MODEL with maps
  note: SPM MOTOR MODEL
  note: INPUTS
  note: OUTPUTS
  uabc : Inport
  tauL : Inport  Port=2
  Clarke + Park 1 : Subsystem
      settings: PortSchema="{\"entries\":[{\"content\":{\"sides\":[{\"content\":{\"connectorIds\":[\"In1\"]},\"type\":\"ConnectorPlacement.EquallySpacedRectSide\",\"uuid\":\"dfbca390-01d3-4350-a1f7-5814b855842b\"},{\"content\":{\"connectorIds\":[\"Out1\"],\"side\":\"RIGHT\"},\"type\":\"ConnectorPlacement.EquallySpacedRectSide\",\"uuid\":\"31b508dd-6a0c-4770-a977-34ff5a62a059\"},{\"content\":{\"connectorIds\":[\"In2\"],\"side\":\"TOP\"},\"type\":\"ConnectorPlacement.EquallySpacedRectSide\",\"uuid\":\"bd902134-125b-49c1-af87-7c7bfb23097c\"},{\"content\":{\"connectorIds\":[],\"side\":\"HIDDEN\"},\"type\":\"ConnectorPlacement.EquallySpacedRectSide\",\"uuid\":\"5c93052a-f73b-4726-be02-ec4253e9ca63\"}]},\"type\":\"ConnectorPlacement.EquallySpacedConnector\",\"uuid\":\"90558e66-2977-4bab-ac0f-d07dc1d3bf9d\"}],\"packageUris\":[\"http://schema.mathworks.com/mf0/Connector/R2020b\"],\"version\":\"1.0\"}"
  Constant : Constant  Value=0
  Gain1 : Gain  Gain=mot.p
  Gain2 : Gain  Gain=mot.p
  Mux : Mux  Inputs=3
  Rev_Park + Rev_Clarke : Subsystem
  SPM Motor : Subsystem
  electrical equations : Subsystem
  mechanical system : Subsystem
      settings: PortSchema="{\"entries\":[{\"content\":{\"sides\":[{\"content\":{\"connectorIds\":[\"In1\",\"In2\",\"In3\",\"In4\"]},\"type\":\"ConnectorPlacement.EquallySpacedRectSide\",\"uuid\":\"ba3eadf5-5339-4096-82c0-65ae6f7654f8\"},{\"content\":{\"connectorIds\":[\"Out1\",\"Out2\",\"Out3\"],\"side\":\"RIGHT\"},\"type\":\"ConnectorPlacement.EquallySpacedRectSide\",\"uuid\":\"5d9f567b-aeb8-4ece-a206-38434530d515\"},{\"content\":{\"connectorIds\":[\"In5\"],\"side\":\"TOP\"},\"type\":\"ConnectorPlacement.EquallySpacedRectSide\",\"uuid\":\"4d5c6e7c-fa05-44b7-bedf-9f7fec742b34\"}]},\"type\":\"ConnectorPlacement.EquallySpacedConnector\",\"uuid\":\"f68f900c-fb94-45c0-a867-bf7e311f1b8e\"}],\"packageUris\":[\"http://schema.mathworks.com/mf0/Connector/19700101\"],\"version\":\"1.0\"}"
  thm : Outport
  wm : Outport  Port=2
  taum : Outport  Port=3
  iabc : Outport  Port=4
  idq : Outport  Port=5
  theta_me : Outport  Port=6
  w_me : Outport  Port=7
  U_A : Outport  Port=8
  U_B : Outport  Port=9
  U_DQ : Outport  Port=10
  wires:
  Rev_Park + Rev_Clarke/1(abc) -> iabc/1
  Clarke + Park 1/1(dq) -> SPM Motor/1(dq)
  SPM Motor/1(theta_me) -> Clarke + Park 1/2(thme)
  Gain1/1 -> w_me/1, [WME]
  Constant/1 -> Mux/3
  [WME] -> electrical equations/3(w_me)
  [THME] -> electrical equations/2(thme)
  [THME] -> Rev_Park + Rev_Clarke/2(thme1)
  Mux/1 -> Rev_Park + Rev_Clarke/1(dq), idq/1
  electrical equations/1(lam_d) -> mechanical system/1(lam_d)
  tauL/1 -> [TAUL], mechanical system/5(tauL)
  uabc/1 -> Clarke + Park 1/1(abc), electrical equations/1(uabc)
  electrical equations/4(id) -> Mux/1, mechanical system/4(id)
  electrical equations/3(iq) -> mechanical system/3(iq), Mux/2
  electrical equations/2(lam_q) -> mechanical system/2(lam_q)
  Gain2/1 -> theta_me/1, [THME]
  SPM Motor/2(w_me) -> ?
  mechanical system/3(wm) -> wm/1, Gain1/1
  mechanical system/1(thm) -> thm/1, Gain2/1
  mechanical system/2(taum) -> taum/1
  electrical equations/5(UA) -> U_A/1
  electrical equations/6(UB) -> U_B/1
  electrical equations/7(UDQ) -> U_DQ/1

== system SalientPolePMSM/DT SENSORLESS ALGORITHM AB/Classic PLL1 ==
  e_alpha : Inport
  e_beta : Inport  Port=2
  In3 : Inport  Port=3
  Cos : Trigonometry  Operator=cos
  Delay{1..4} (4 alike) : Delay  DelayLength=1  SampleTime=Obs.Ts
  Discrete Filter1 : DiscreteFilter  Numerator=[Obs.lpf.alpha*3]  Denominator=[1 ((Obs.lpf.alpha*3)-1)]  SampleTime=Obs.Ts
  Discrete PID Controller : pid_lib/PID Controller  Controller=PID  Form=Parallel  TimeDomain=Discrete-time  UseExternalTs=off  SampleTime=Obs.Ts  IntegratorMethod=Forward Euler  FilterMethod=Forward Euler  ControllerParametersSource=internal  P=0.05  I=Obs.PI.ki*Obs.Ts  D=0  UseFilter=off  N=100  TunerSelectOption=Transfer Function Based (PID Tuner App)  ZeroCross=off  InitialConditionSource=internal  InitialConditionForIntegrator=0  InitialConditionForFilter=0  DifferentiatorICPrevScaledInput=0  ExternalReset=none  TrackingMode=off  Kt=1  LimitOutput=off  SatLimitsSource=internal  UpperSaturationLimit=inf  LowerSaturationLimit=-inf  LinearizeAsGain=off  AntiWindupMode=none  Kb=1  POutMin=[]  POutMax=[]  IOutMin=[]  IOutMax=[]  DOutMin=[]  DOutMax=[]  NOutMin=[]  NOutMax=[]  SumOutMin=[]  SumOutMax=[]  SaturationOutMin=[]  SaturationOutMax=[]  PParamMin=[]  PParamMax=[]  IParamMin=[]  IParamMax=[]  DParamMin=[]  DParamMax=[]  NParamMin=[]  NParamMax=[]  KbParamMin=[]  KbParamMax=[]  KtParamMin=[]  KtParamMax=[]  KbOutMin=[]  KbOutMax=[]  KtOutMin=[]  KtOutMax=[]  IntegratorOutMin=[]  IntegratorOutMax=[]  FilterOutMin=[]  FilterOutMax=[]  SumI1OutMin=[]  SumI1OutMax=[]  SumI2OutMin=[]  SumI2OutMax=[]  SumI3OutMin=[]  SumI3OutMax=[]  SumI4OutMin=[]  SumI4OutMax=[]  SumDOutMin=[]  SumDOutMax=[]  DifferentiatorOutMin=[]  DifferentiatorOutMax=[]  FilterDiffOutCoefMin=[]  FilterDiffOutCoefMax=[]  ReciprocalOutMin=[]  ReciprocalOutMax=[]  SumDenOutMin=[]  SumDenOutMax=[]  SumNumOutMin=[]  SumNumOutMax=[]  DivideOutMin=[]  DivideOutMax=[]  UdiffTsProdOutMin=[]  UdiffTsProdOutMax=[]  NTsProdOutMin=[]  NTsProdOutMax=[]  UintegralTsProdOutMin=[]  UintegralTsProdOutMax=[]  UngainTsProdOutMin=[]  UngainTsProdOutMax=[]  IntegratorContinuousStateAttributes=''  IntegratorStateMustResolveToSignalObject=off  IntegratorRTWStateStorageClass=Auto  FilterContinuousStateAttributes=''  FilterStateMustResolveToSignalObject=off  FilterRTWStateStorageClass=Auto  ParallelPVariant=InternalParameters  IdealPVariant=Disabled  IVariant=InternalParameters  DVariant=InternalParameters  IntegratorVariant=Discrete  SatVariant=Disabled  AWVariant=Passthrough  PCopyVariant=Disabled  TRVariant=Disabled  FdbkBlocksVariant=Forward  IdealPFdbkVariant=Disabled  SatFdbkVariant=Disabled  DerivativeFilterVariant=Differentiator  NVariant=Passthrough  NCopyVariant=Disabled_SignalSpec  FilterICVariant=InternalICsDifferentiator  IntegratorICVariant=InternalICs  ExternalResetVariant=Disabled  TRSumVariant=Passthrough  SumFdbkVariant=Disabled  SumVariant=Sum_PID  TsampFilterVariant=InternalTs  TsampNgainVariant=Passthrough  TsampIntegralVariant=Passthrough  ExternalSaturationOutDataTypeStr=Inherit: Same as second input
  Discrete PID Controller1 : pid_lib/PID Controller  Controller=PID  Form=Parallel  TimeDomain=Discrete-time  UseExternalTs=off  SampleTime=Obs.Ts  IntegratorMethod=Forward Euler  FilterMethod=Forward Euler  ControllerParametersSource=internal  P=1  I=0.1  D=0  UseFilter=off  N=100  TunerSelectOption=Transfer Function Based (PID Tuner App)  ZeroCross=off  InitialConditionSource=internal  InitialConditionForIntegrator=0  InitialConditionForFilter=0  DifferentiatorICPrevScaledInput=0  ExternalReset=none  TrackingMode=off  Kt=1  LimitOutput=off  SatLimitsSource=internal  UpperSaturationLimit=inf  LowerSaturationLimit=-inf  LinearizeAsGain=off  AntiWindupMode=none  Kb=1  POutMin=[]  POutMax=[]  IOutMin=[]  IOutMax=[]  DOutMin=[]  DOutMax=[]  NOutMin=[]  NOutMax=[]  SumOutMin=[]  SumOutMax=[]  SaturationOutMin=[]  SaturationOutMax=[]  PParamMin=[]  PParamMax=[]  IParamMin=[]  IParamMax=[]  DParamMin=[]  DParamMax=[]  NParamMin=[]  NParamMax=[]  KbParamMin=[]  KbParamMax=[]  KtParamMin=[]  KtParamMax=[]  KbOutMin=[]  KbOutMax=[]  KtOutMin=[]  KtOutMax=[]  IntegratorOutMin=[]  IntegratorOutMax=[]  FilterOutMin=[]  FilterOutMax=[]  SumI1OutMin=[]  SumI1OutMax=[]  SumI2OutMin=[]  SumI2OutMax=[]  SumI3OutMin=[]  SumI3OutMax=[]  SumI4OutMin=[]  SumI4OutMax=[]  SumDOutMin=[]  SumDOutMax=[]  DifferentiatorOutMin=[]  DifferentiatorOutMax=[]  FilterDiffOutCoefMin=[]  FilterDiffOutCoefMax=[]  ReciprocalOutMin=[]  ReciprocalOutMax=[]  SumDenOutMin=[]  SumDenOutMax=[]  SumNumOutMin=[]  SumNumOutMax=[]  DivideOutMin=[]  DivideOutMax=[]  UdiffTsProdOutMin=[]  UdiffTsProdOutMax=[]  NTsProdOutMin=[]  NTsProdOutMax=[]  UintegralTsProdOutMin=[]  UintegralTsProdOutMax=[]  UngainTsProdOutMin=[]  UngainTsProdOutMax=[]  IntegratorContinuousStateAttributes=''  IntegratorStateMustResolveToSignalObject=off  IntegratorRTWStateStorageClass=Auto  FilterContinuousStateAttributes=''  FilterStateMustResolveToSignalObject=off  FilterRTWStateStorageClass=Auto  ParallelPVariant=InternalParameters  IdealPVariant=Disabled  IVariant=InternalParameters  DVariant=InternalParameters  IntegratorVariant=Discrete  SatVariant=Disabled  AWVariant=Passthrough  PCopyVariant=Disabled  TRVariant=Disabled  FdbkBlocksVariant=Forward  IdealPFdbkVariant=Disabled  SatFdbkVariant=Disabled  DerivativeFilterVariant=Differentiator  NVariant=Passthrough  NCopyVariant=Disabled_SignalSpec  FilterICVariant=InternalICsDifferentiator  IntegratorICVariant=InternalICs  ExternalResetVariant=Disabled  TRSumVariant=Passthrough  SumFdbkVariant=Disabled  SumVariant=Sum_PID  TsampFilterVariant=InternalTs  TsampNgainVariant=Passthrough  TsampIntegralVariant=Passthrough  ExternalSaturationOutDataTypeStr=Inherit: Same as second input
  Discrete-Time Integrator : DiscreteIntegrator  SampleTime=Obs.Ts  ICPrevOutput=DiscIntNeverNeededParam  ICPrevScaledInput=DiscIntNeverNeededParam
  Divide1 : Product  Inputs=**
  Divide2 : Product  Inputs=**
  MATLAB Function1 : MATLAB Function  TreatAsAtomicUnit=on
  MATLAB Function2 : MATLAB Function  TreatAsAtomicUnit=on
  Scope{,1..3} (4 alike) : Scope  NumInputPorts=2
  Sin : Trigonometry
  Sum : Sum  Inputs=+|-
  thme_est1 : Outport
  wme_est1 : Outport  Port=2
  wires:
  e_beta/1 -> Scope2/2, Delay1/1
  e_alpha/1 -> Scope2/1, Delay2/1
  Delay2/1 -> Divide1/1
  Divide1/1 -> Scope/1, Sum/1
  Divide2/1 -> Scope/2, Sum/2
  Delay1/1 -> Divide2/1
  Sin/1 -> Divide2/2
  Cos/1 -> Divide1/2
  Delay4/1 -> Sin/1
  Delay3/1 -> Cos/1
  Sum/1 -> Discrete PID Controller1/1, Scope1/2
  Discrete-Time Integrator/1 -> Delay4/1, Delay3/1, Scope3/1, thme_est1/1
  In3/1 -> Scope3/2
  Discrete Filter1/1 -> wme_est1/1
  Discrete PID Controller1/1 -> MATLAB Function2/1(u)
  MATLAB Function2/1(y) -> Discrete Filter1/1, Discrete-Time Integrator/1

== system SalientPolePMSM/DT SENSORLESS ALGORITHM AB/Normalized and improved PLL2 ==
  e_d : Inport
  e_q : Inport  Port=2
  Cos : Trigonometry  Operator=cos
  Delay{1..4} (4 alike) : Delay  DelayLength=1  SampleTime=Obs.Ts
  Discrete Filter1 : DiscreteFilter  Commented=on  Numerator=[dqpll.lpf.alpha]  Denominator=[1 (dqpll.lpf.alpha-1)]
  Discrete PI : Subsystem
  Discrete-Time Integrator : DiscreteIntegrator  SampleTime=Obs.Ts  ICPrevOutput=DiscIntNeverNeededParam  ICPrevScaledInput=DiscIntNeverNeededParam
  Divide1 : Product  Inputs=**
  Divide2 : Product  Inputs=**
  Divide3 : Product  Inputs=**
  Gain : Gain  Gain=-2
  Gain1 : Gain  Gain=0.5
  Gain2 : Gain  Gain=2
  Gain3 : Gain  Gain=2
  Power of 1 : Math  Operator=magnitude^2  SaturateOnIntegerOverflow=on
  Power of 10 : Math  Operator=magnitude^2  SaturateOnIntegerOverflow=on
  Scope : Scope  NumInputPorts=2
  Sin : Trigonometry
  Sum : Sum  Inputs=-|+
  Sum1 : Sum  Inputs=|+-
  thme_est1 : Outport
  wme_est1 : Outport  Port=2
  wires:
  e_d/1 -> Delay2/1
  Divide1/1 -> Scope/1, Sum/1
  Divide2/1 -> Scope/2, Sum/2
  Sin/1 -> Divide2/2
  Cos/1 -> Divide1/2
  Discrete-Time Integrator/1 -> thme_est1/1, Delay3/1, Delay4/1
  Discrete PI/1(w_est) -> wme_est1/1, Discrete-Time Integrator/1
  Gain/1 -> Divide3/1
  Divide3/1 -> Divide2/1
  e_q/1 -> Delay1/1
  Power of 1/1 -> Sum1/1
  Power of 10/1 -> Sum1/2
  Sum1/1 -> Divide1/1
  Sum/1 -> Gain1/1
  Gain1/1 -> Discrete PI/1(e)
  Gain3/1 -> Sin/1
  Gain2/1 -> Cos/1
  Delay2/1 -> Gain/1, Power of 1/1
  Delay1/1 -> Divide3/2, Power of 10/1
  Delay3/1 -> Gain3/1
  Delay4/1 -> Gain2/1

== system SalientPolePMSM/DT SENSORLESS ALGORITHM AB/Observer ==
  u(k) : Inport
  y(k) : Inport  Port=2
  Demux : Demux
  Gain : Gain  Gain=Obs.G
  Gain1 : Gain  Gain=Obs.C
  Gain2 : Gain  Gain=Obs.F
  Gain3 : Gain  Gain=Obs.K
  Gain4 : Gain  Gain=Obs.G
  Sum : Sum  Inputs=|-+
  Sum1 : Sum  Inputs=+++
  Terminator : Terminator
  Terminator1 : Terminator
  e_alpha : Outport
  e_beta : Outport  Port=2
  wires:
  u(k)/1 -> Gain/1
  Demux/3 -> e_alpha/1
  Demux/4 -> e_beta/1
  Demux/2 -> Terminator/1
  Demux/1 -> Terminator1/1
  Gain4/1 -> Demux/1, Gain2/1, Gain1/1  "x_est(k)"
  Gain/1 -> Sum1/2
  Gain2/1 -> Sum1/3
  Gain1/1 -> Sum/1  "y_est(k)"
  y(k)/1 -> Sum/2
  Sum/1 -> Gain3/1
  Gain3/1 -> Sum1/1
  Sum1/1 -> Gain4/1
